simulink model "springdamper_t"  (R2018a)
settings: Solver=VariableStepAuto  StartTime=0.0  StopTime=100  RelTol=1e-3
settings Model: Creator=Administrator  LastModifiedBy=Administrator

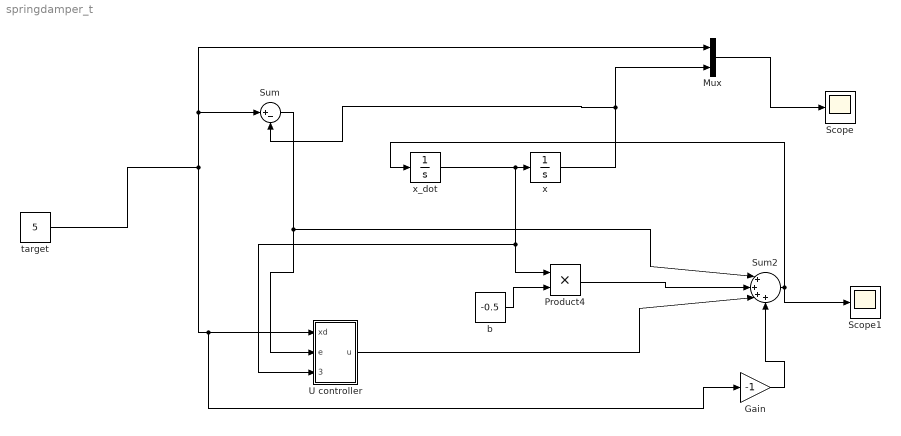
== system springdamper_t ==
  Gain : Gain  Gain=-1
  Mux : Mux  Inputs=2
  Product4 : Product
  Scope : Scope
  Scope1 : Scope
  Sum : Sum  Inputs=|+-
  Sum2 : Sum  Inputs=|++++
  U controller : Subsystem
  b : Constant  Value=-0.5
  target : Constant  Value=5
  x : Integrator
  x_dot : Integrator
  wires:
  x_dot/1 -> U controller/3(xdot), Product4/1, x/1
  x/1 -> Mux/2, Sum/2
  Sum/1 -> U controller/2(e), Sum2/1
  b/1 -> Product4/2
  Sum2/1 -> Scope1/1, x_dot/1
  Gain/1 -> Sum2/4
  Product4/1 -> Sum2/2
  U controller/1(u) -> Sum2/3
  target/1 -> Sum/1, Mux/1, U controller/1(xd), Gain/1
  Mux/1 -> Scope/1

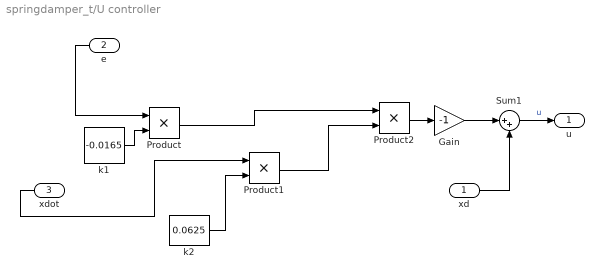
== system springdamper_t/U controller ==
  xd : Inport
  e : Inport  Port=2
  xdot : Inport  Port=3
  Gain : Gain  Gain=-1
  Product : Product
  Product1 : Product
  Product2 : Product
  Sum1 : Sum  Inputs=|++
  k1 : Constant  Value=-0.0165
  k2 : Constant  Value=0.0625
  u : Outport
  wires:
  k1/1 -> Product/2
  Product1/1 -> Product2/2
  Product2/1 -> Gain/1
  Gain/1 -> Sum1/1
  e/1 -> Product/1
  xd/1 -> Sum1/2
  Sum1/1 -> u/1  "u"
  Product/1 -> Product2/1
  k2/1 -> Product1/2
  xdot/1 -> Product1/1
